simulink model "followerController_exp4"  (R2016a)
settings: Solver=FixedStepAuto  StartTime=0.0  StopTime=inf  RelTol=1e-3
undefined symbols (not defined in the file or in its folder): Angular, Linear
libraries: robotlib x7
settings Model: Creator=ece446  LastModifiedBy=ece446
settings OptimizationCC: OptimizeModelRefInitCode=on  LifeSpan=Inf  MaxStackSize=64
settings HardwareCC: ProdBitPerInt=16  ProdBitPerPointer=16  ProdLargestAtomicFloat=None  ProdIntDivRoundTo=Undefined  ProdEndianess=Unspecified  ProdWordSize=16  ProdHWDeviceType=Generic->Unspecified (assume 32-bit Generic)  UseEmbeddedCoderFeatures=off
settings RTWCC: SystemTargetFile=ert.tlc  HardwareBoard=Robot Operating System (ROS)  TemplateMakefile=ert_default_tmf  GenerateReport=on  Toolchain=Catkin  IncludeHyperlinkInReport=on  LaunchReport=on  TargetLang=C++  GenerateTraceInfo=on  GenerateTraceReport=on  GenerateTraceReportSl=on  GenerateTraceReportSf=on  GenerateTraceReportEml=on
settings CodeAppCC: ForceParamTrailComments=on  IgnoreCustomStorageClasses=off  OperatorAnnotations=on  SimulinkDataObjDesc=on  SFDataObjDesc=on  MATLABFcnDesc=on  InsertBlockDesc=on  MATLABSourceComments=on
settings ERTTargetCC: SupportNonInlinedSFcns=on

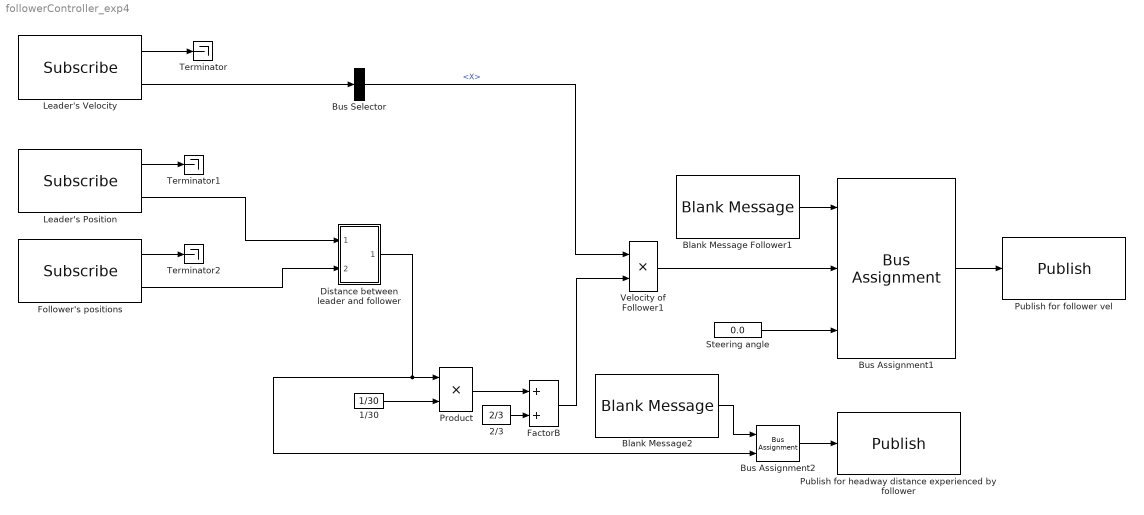
== system followerController_exp4 ==
  1/30 : Constant  Value=1/30
  2/3 : Constant  Value=2/3
  Blank Message Follower1 : robotlib/Blank Message  SourceLibraryInfo=This block requires Robotics System Toolbox  messageType=geometry_msgs/Twist  SampleTime=inf
  Blank Message2 : robotlib/Blank Message  SourceLibraryInfo=This block requires Robotics System Toolbox  messageType=std_msgs/Float64  SampleTime=inf
  Bus Assignment1 : BusAssignment  AssignedSignals=Linear.X,Angular.Z
  Bus Assignment2 : BusAssignment  AssignedSignals=Data
  Bus Selector : BusSelector  OutputSignals=Linear.X
  Distance between leader and follower : Subsystem
  FactorB : Sum
  Follower's positions : robotlib/Subscribe  SourceLibraryInfo=This block requires Robotics System Toolbox  topicSource=Select from ROS network  topic=/follower_sim/odom  messageType=nav_msgs/Odometry  sampleTime=-1  messageQueueLength=1
  Leader's Position : robotlib/Subscribe  SourceLibraryInfo=This block requires Robotics System Toolbox  topicSource=Select from ROS network  topic=/azcar_sim/odom  messageType=nav_msgs/Odometry  sampleTime=-1  messageQueueLength=1
  Leader's Velocity : robotlib/Subscribe  SourceLibraryInfo=This block requires Robotics System Toolbox  topicSource=Select from ROS network  topic=/azcar_sim/vel  messageType=geometry_msgs/Twist  sampleTime=-1  messageQueueLength=1
  Product : Product
  Publish for follower vel : robotlib/Publish  SourceLibraryInfo=This block requires Robotics System Toolbox  topicSource=Select from ROS network  topic=/follower_sim/cmd_vel  messageType=geometry_msgs/Twist  messageQueueLength=1
  Publish for headway distance experienced by follower : robotlib/Publish  SourceLibraryInfo=This block requires Robotics System Toolbox  topicSource=Specify your own  topic=/follower_sim/headway  messageType=std_msgs/Float64  messageQueueLength=1
  Steering angle : Constant  Value=0.0
  Terminator : Terminator
  Terminator1 : Terminator
  Terminator2 : Terminator
  Velocity of Follower1 : Product
  wires:
  1/30/1 -> Product/2
  Product/1 -> FactorB/1
  2/3/1 -> FactorB/2
  Blank Message Follower1/1 -> Bus Assignment1/1
  Bus Assignment1/1 -> Publish for follower vel/1
  Velocity of Follower1/1 -> Bus Assignment1/2
  FactorB/1 -> Velocity of Follower1/2
  Steering angle/1 -> Bus Assignment1/3
  Leader's Velocity/2 -> Bus Selector/1
  Leader's Velocity/1 -> Terminator/1
  Bus Selector/1 -> Velocity of Follower1/1  "<X>"
  Leader's Position/1 -> Terminator1/1
  Follower's positions/1 -> Terminator2/1
  Leader's Position/2 -> Distance between leader and follower/1(In1)
  Follower's positions/2 -> Distance between leader and follower/2(In2)
  Bus Assignment2/1 -> Publish for headway distance experienced by follower/1
  Blank Message2/1 -> Bus Assignment2/1
  Distance between leader and follower/1(Out1) -> Product/1, Bus Assignment2/2

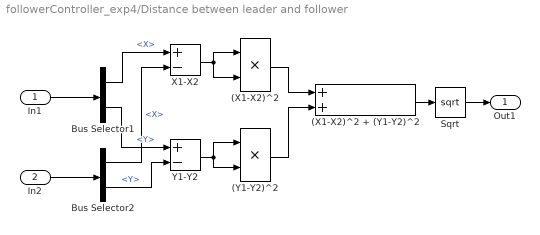
== system followerController_exp4/Distance between leader and follower ==
  In1 : Inport
  In2 : Inport  Port=2
  (X1-X2)^2 : Product
  (X1-X2)^2 + (Y1-Y2)^2 : Sum
  (Y1-Y2)^2 : Product
  Bus Selector1 : BusSelector  OutputSignals=Pose.Pose.Position.X,Pose.Pose.Position.Y
  Bus Selector2 : BusSelector  OutputSignals=Pose.Pose.Position.X,Pose.Pose.Position.Y
  Sqrt : Sqrt  SaturateOnIntegerOverflow=on
  X1-X2 : Sum  Inputs=+-
  Y1-Y2 : Sum  Inputs=+-
  Out1 : Outport
  wires:
  Bus Selector1/1 -> X1-X2/1  "<X>"
  Bus Selector2/2 -> Y1-Y2/2  "<Y>"
  (Y1-Y2)^2/1 -> (X1-X2)^2 + (Y1-Y2)^2/2
  (X1-X2)^2 + (Y1-Y2)^2/1 -> Sqrt/1
  (X1-X2)^2/1 -> (X1-X2)^2 + (Y1-Y2)^2/1
  Bus Selector1/2 -> Y1-Y2/1  "<Y>"
  In1/1 -> Bus Selector1/1
  Bus Selector2/1 -> X1-X2/2  "<X>"
  Y1-Y2/1 -> (Y1-Y2)^2/2, (Y1-Y2)^2/1
  X1-X2/1 -> (X1-X2)^2/2, (X1-X2)^2/1
  Sqrt/1 -> Out1/1
  In2/1 -> Bus Selector2/1
